simulink model "Load_Cell_Simulink"  (R2020a)
settings: Solver=VariableStepAuto  StartTime=0.0  StopTime=10  RelTol=1e-3
libraries: fl_lib x19, ee_lib x12, nesl_utility x7, simulink x1
settings Model: Creator=parsa  LastModifiedBy=parsa

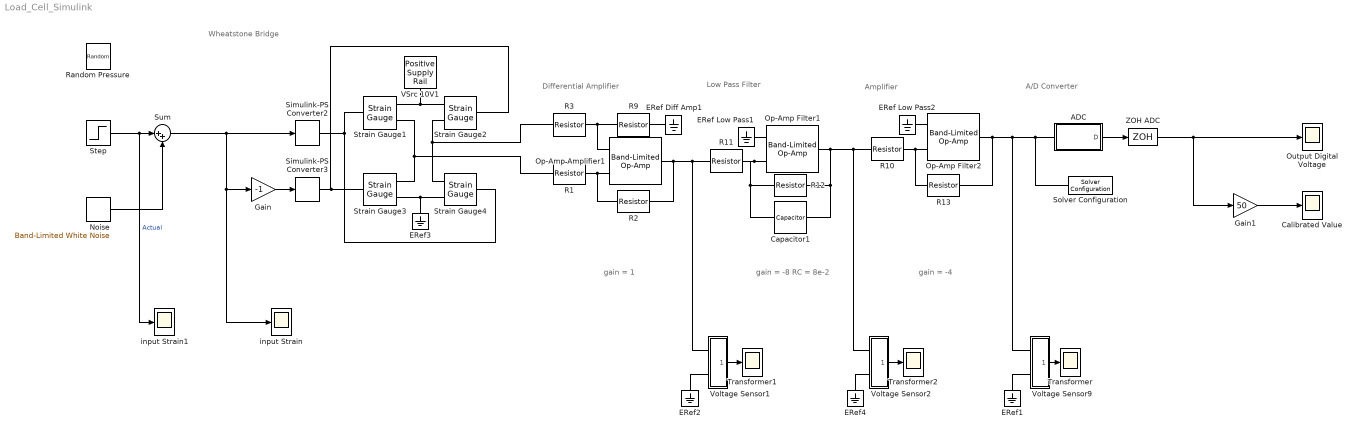
== system Load_Cell_Simulink ==
  note: A/D Converter
  note: Amplifier
  note: gain = -8
      | RC = 8e-2
  note: Low Pass Filter
  note: Wheatstone Bridge
  note: gain = 1
  note: Differential Amplifier
  note: gain = -4
  ADC : Subsystem  mask(ADC){N=24, vmax=9, ileak=1e-9, C=10e-12}
      mask prompts: N "Number of bits"; vmax "Input voltage for max output (V)"; ileak "Leakage current (A)"; C "Pin capacitance (F)"
      mask help: Simplified analog-to-digital converter
  Calibrated Value : Scope
  Capacitor1 : ee_lib/Passive/Capacitor  cap_option=0  c=10e-6 F  Cvec=[ 1e-5 1e-6 ] F  Vvec=[ 0 10 ] V  CV_table_symmetry=1  f_vec=[1, 10] kHz  DFext_vec=[.8, 1.2]  C_tol=5  enable_C_tol=0  tol_distribution=1  nSigma=4  r=1e-6 Ohm  g=0 1/Ohm  averaging_period=0 s  enable_operating_limits=0  operating_limit_action=2  max_working_voltage_range=[ -25 25 ] V  power_rating=1 W  enable_faults=0  fault_action=1  Cscale_faulted=100  R_faulted=0.001 Ohm  G_faulted=0 1/Ohm  tau_fault=0.001 s  enable_temporal_fault=0  t_fault=1 s  enable_behavioral_fault=0  max_permissible_voltage_range=[ -100 100 ] V  t_fail_on_voltage=1 s  i_specify=off  i_priority=None  i=0 A  i_nominal_specify=off  i_nominal_unit=A  i_nominal_value=1  v_specify=off  v_priority=None  v=0 V  v_nominal_specify=off  v_nominal_unit=V  v_nominal_value=1  vc_specify=on  vc_priority=High  vc=0 V  vc_nominal_specify=off  vc_nominal_unit=V  vc_nominal_value=1
  ERef Diff Amp1 : fl_lib/Electrical/Electrical Elements/Electrical Reference
      settings: SourceProductBaseCode=MT,SS
  ERef Low Pass1 : fl_lib/Electrical/Electrical Elements/Electrical Reference
      settings: SourceProductBaseCode=MT,SS
  ERef Low Pass2 : fl_lib/Electrical/Electrical Elements/Electrical Reference
      settings: SourceProductBaseCode=MT,SS
  ERef{1..4} (4 alike) : fl_lib/Electrical/Electrical Elements/Electrical Reference
  Gain : Gain  Gain=-1
  Gain1 : Gain  Gain=50
  Noise : simulink/Sources/Band-Limited White Noise  Cov=1e-10  Ts=0.001  seed=[23341]
  Op-Amp Amplifier1 : ee_lib/Integrated Circuits/Band-Limited Op-Amp  A=1000  Rin=1e+06 Ohm  Rout=100 Ohm  Vmin=-15 V  Vmax=15 V  Vdotmax=1000 V/s  f=1e5 Hz  V0=0 V
      settings: SourceProductBaseCode=PS
  Op-Amp Filter1 : ee_lib/Integrated Circuits/Band-Limited Op-Amp  A=1000  Rin=1e+06 Ohm  Rout=100 Ohm  Vmin=-15 V  Vmax=15 V  Vdotmax=1000 V/s  f=1e5 Hz  V0=0 V
      settings: SourceProductBaseCode=PS
  Op-Amp Filter2 : ee_lib/Integrated Circuits/Band-Limited Op-Amp  A=1000  Rin=1e+06 Ohm  Rout=100 Ohm  Vmin=-15 V  Vmax=15 V  Vdotmax=1000 V/s  f=1e5 Hz  V0=0 V
      settings: SourceProductBaseCode=PS
  Output Digital Voltage : Scope
  R{1..3,9} (4 alike) : fl_lib/Electrical/Electrical Elements/Resistor  R=10 kOhm  i_specify=off  i_priority=High  i=0 A  i_nominal_specify=off  i_nominal_unit=A  i_nominal_value=1  v_specify=off  v_priority=High  v=0 V  v_nominal_specify=off  v_nominal_unit=V  v_nominal_value=1
      settings: SourceProductBaseCode=MT,SS
  R10 : ee_lib/Passive/Resistor  R=1 kOhm  R_tol=5  enable_R_tol=0  tol_distribution=1  nSigma=4  enable_operating_limits=0  operating_limit_action=2  max_working_voltage=100 V  power_rating=1 W  enable_faults=0  fault_action=1  R_faulted=Inf Ohm  enable_temporal_fault=0  t_fault=1 s  enable_behavioral_fault=0  max_permissible_current=1 A  t_fail_on_current=1 s  noise_mode=0  sample_time=0.001 s  repeatability=1  auto_seed=2639802684  user_seed=0  Tdevice=25 degC  alpha=3.93e-3 1/K  Tmeas=25 degC  thermal_mass=100 J/K  power_derating_T1=70 degC  power_derating_T2=155 degC  operating_temperature_range_vec=[-50, 150] degC  temperature_specify=off  temperature_priority=High  temperature=298.15 K  temperature_nominal_specify=off  temperature_nominal_unit=K  temperature_nominal_value=1
  R11 : fl_lib/Electrical/Electrical Elements/Resistor  R=1 kOhm  i_specify=off  i_priority=High  i=0 A  i_nominal_specify=off  i_nominal_unit=A  i_nominal_value=1  v_specify=off  v_priority=High  v=0 V  v_nominal_specify=off  v_nominal_unit=V  v_nominal_value=1
      settings: SourceProductBaseCode=MT,SS
  R12 : ee_lib/Passive/Resistor  R=8 kOhm  R_tol=5  enable_R_tol=0  tol_distribution=1  nSigma=4  enable_operating_limits=0  operating_limit_action=2  max_working_voltage=100 V  power_rating=1 W  enable_faults=0  fault_action=1  R_faulted=Inf Ohm  enable_temporal_fault=0  t_fault=1 s  enable_behavioral_fault=0  max_permissible_current=1 A  t_fail_on_current=1 s  noise_mode=0  sample_time=0.001 s  repeatability=1  auto_seed=47154843  user_seed=0  Tdevice=25 degC  alpha=3.93e-3 1/K  Tmeas=25 degC  thermal_mass=100 J/K  power_derating_T1=70 degC  power_derating_T2=155 degC  operating_temperature_range_vec=[-50, 150] degC  temperature_specify=off  temperature_priority=High  temperature=298.15 K  temperature_nominal_specify=off  temperature_nominal_unit=K  temperature_nominal_value=1
  R13 : ee_lib/Passive/Resistor  R=4 kOhm  R_tol=5  enable_R_tol=0  tol_distribution=1  nSigma=4  enable_operating_limits=0  operating_limit_action=2  max_working_voltage=100 V  power_rating=1 W  enable_faults=0  fault_action=1  R_faulted=Inf Ohm  enable_temporal_fault=0  t_fault=1 s  enable_behavioral_fault=0  max_permissible_current=1 A  t_fail_on_current=1 s  noise_mode=0  sample_time=0.001 s  repeatability=1  auto_seed=2462134598  user_seed=0  Tdevice=25 degC  alpha=3.93e-3 1/K  Tmeas=25 degC  thermal_mass=100 J/K  power_derating_T1=70 degC  power_derating_T2=155 degC  operating_temperature_range_vec=[-50, 150] degC  temperature_specify=off  temperature_priority=High  temperature=298.15 K  temperature_nominal_specify=off  temperature_nominal_unit=K  temperature_nominal_value=1
  "Random Pressure " : UniformRandomNumber  Minimum=0  Maximum=1e-4  SampleTime=2
  Simulink-PS Converter2 : nesl_utility/Simulink-PS Converter  PhysicalDomain=network_engine_domain  SubClassName=ps_input  LeftPortType=input  RightPortType=output  PseudoPeriodic=off  Frequencies=[]  NoiseDistribution=none  NoiseParameters=[]  Unit=1  AffineConversion=off  FilteringAndDerivatives=zero  SimscapeFilterOrder=1  InputFilterTimeConstant=.001  UdotUserProvided=0
      settings: SourceProductBaseCode=MT,SS
  Simulink-PS Converter3 : nesl_utility/Simulink-PS Converter  PhysicalDomain=network_engine_domain  SubClassName=ps_input  LeftPortType=input  RightPortType=output  PseudoPeriodic=off  Frequencies=[]  NoiseDistribution=none  NoiseParameters=[]  Unit=1  AffineConversion=off  FilteringAndDerivatives=zero  SimscapeFilterOrder=1  InputFilterTimeConstant=.001  UdotUserProvided=0
      settings: SourceProductBaseCode=MT,SS
  Solver Configuration : nesl_utility/Solver Configuration  PhysicalDomain=network_engine_domain  SubClassName=solver  LeftPortType=input  RightPortType=generic  Tones=[]  Harmonics=[]  SimulateNoise=off  Profile=off  UseLocalSampling=off  EnableSwitchedLinearOptims=on  FrequencyDomain=off  UseCCode=off  RelTol=0.001  AbsTol=1e-06  MinStep=1e-09  ToWorkspace=off  RevertToSquareIcSolve=off  NumHomotopyIterations=100  PhasorMode=off  PhasorModeNumHarmonics=1  DoDC=off  ResidualTolerance=1e-09  UseLocalSolver=off  LocalSolverChoice=NE_BACKWARD_EULER_ADVANCER  LocalSolverSampleTime=0.001  DoFixedCost=off  MaxNonlinIter=3  MaxModeIter=2  LinearAlgebra=Sparse  EquationFormulation=NE_TIME_EF  DelaysMemoryBudget=1024  AutomaticFiltering=on  FilteringTimeConstant=0.001  PartitionStorageMethod=AS_NEEDED  PartitionMemoryBudget=1024  PartitionMethod=FAST
  Step : Step  After=1e-4  SampleTime=0
  Strain Gauge{1..4} (4 alike) : ee_lib/Sensors & Transducers/Strain Gauge  R=100 Ohm  K=2
      settings: SourceProductBaseCode=PS  InternalSimscapePortConfiguration="{\"Bottom\":[],\"Left\":[{\"id\":\"E\",\"label\":\"E\",\"type\":\"input\"}],\"Right\":[{\"id\":\"p\",\"label\":\"+\",\"type\":\"foundation.electrical.electrical\"},{\"id\":\"n\",\"label\":\"-\",\"type\":\"foundation.electrical.electrical\"}],\"Top\":[]}"
  Sum : Sum  Inputs=|++
  Transformer : Scope
  Transformer1 : Scope
  Transformer2 : Scope
  VSrc 10V1 : ee_lib/Sources/Positive Supply Rail  v0=9 V
      settings: SourceProductBaseCode=PS  InternalSimscapePortConfiguration="{\"Bottom\":[],\"Left\":[],\"Right\":[{\"id\":\"p\",\"label\":\"\",\"type\":\"foundation.electrical.electrical\"}],\"Top\":[]}"
  Voltage Sensor1 : Subsystem
  Voltage Sensor2 : Subsystem
  Voltage Sensor9 : Subsystem
  ZOH ADC : ZeroOrderHold  SampleTime=0.01
  input Strain : Scope
  input Strain1 : Scope
  wires:
  Gain/1 -> Simulink-PS Converter3/1
  ADC/1(D) -> ZOH ADC/1
  Voltage Sensor9/1(V) -> Transformer/1
  Voltage Sensor1/1(V) -> Transformer1/1
  Voltage Sensor2/1(V) -> Transformer2/1
  ZOH ADC/1 -> Gain1/1, Output Digital Voltage/1
  Gain1/1 -> Calibrated Value/1
  Noise/1 -> Sum/2
  Step/1 -> input Strain1/1, Sum/1  "Actual"
  Sum/1 -> input Strain/1, Gain/1, Simulink-PS Converter2/1
  connections:
  Op-Amp Filter2/LConn2 -- R10/RConn1 -- R13/LConn1
  Strain Gauge4/RConn2 -- Strain Gauge3/RConn2 -- ERef3/LConn1
  R3/LConn1 -- Strain Gauge4/RConn1 -- Strain Gauge2/RConn2
  Strain Gauge3/LConn1 -- Strain Gauge2/LConn1 -- Simulink-PS Converter3/RConn1
  R2/LConn1 -- Op-Amp Amplifier1/LConn2 -- R1/RConn1
  R1/LConn1 -- Strain Gauge1/RConn2 -- Strain Gauge3/RConn1
  Op-Amp Filter2/RConn1 -- R13/RConn1 -- Voltage Sensor9/LConn1 -- ADC/LConn1 -- Solver Configuration/RConn1
  Capacitor1/LConn1 -- R12/LConn1 -- R11/RConn1 -- Op-Amp Filter1/LConn2
  Capacitor1/RConn1 -- R12/RConn1 -- R10/LConn1 -- Voltage Sensor2/LConn1 -- Op-Amp Filter1/RConn1
  R2/RConn1 -- R11/LConn1 -- Voltage Sensor1/LConn1 -- Op-Amp Amplifier1/RConn1
  Strain Gauge1/RConn1 -- Strain Gauge2/RConn1 -- VSrc 10V1/RConn1
  Strain Gauge4/LConn1 -- Simulink-PS Converter2/RConn1 -- Strain Gauge1/LConn1
  R9/LConn1 -- R3/RConn1 -- Op-Amp Amplifier1/LConn1
  ERef Low Pass2/LConn1 -- Op-Amp Filter2/LConn1
  ERef Low Pass1/LConn1 -- Op-Amp Filter1/LConn1
  ERef Diff Amp1/LConn1 -- R9/RConn1
  ERef1/LConn1 -- Voltage Sensor9/LConn2
  ERef2/LConn1 -- Voltage Sensor1/LConn2
  ERef4/LConn1 -- Voltage Sensor2/LConn2

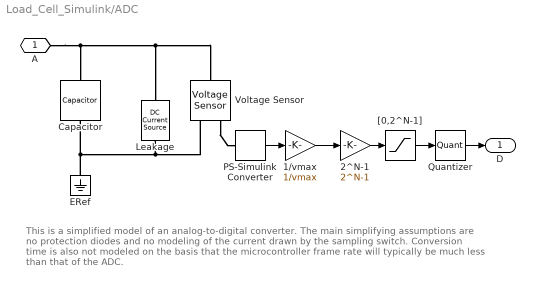
== system Load_Cell_Simulink/ADC ==
  note: This is a simplified model of an analog-to-digital converter. The main simplifying assumptions
      | are no protection diodes and no modeling of the current drawn by the sampling switch.
      | Conversion time is also not modeled on the basis that the microcontroller frame rate will
      | typically be much less than that of the ADC.
  1/vmax : Gain  Gain=1/vmax
  2^N-1 : Gain  Gain=2^N-1
  Capacitor : fl_lib/Electrical/Electrical Elements/Capacitor  c=1e-6 F  r=1e-6 Ohm  g=0 1/Ohm  i_specify=off  i_priority=High  i=0 A  i_nominal_specify=off  i_nominal_unit=A  i_nominal_value=1  v_specify=off  v_priority=High  v=0 V  v_nominal_specify=off  v_nominal_unit=V  v_nominal_value=1  vc_specify=on  vc_priority=High  vc=0 V  vc_nominal_specify=off  vc_nominal_unit=V  vc_nominal_value=1
      settings: SourceProductBaseCode=MT,SS
  ERef : fl_lib/Electrical/Electrical Elements/Electrical Reference
      settings: SourceProductBaseCode=MT,SS
  Leakage : fl_lib/Electrical/Electrical Sources/DC Current Source  i0=ileak A
      settings: SourceProductBaseCode=MT,SS  InternalSimscapePortConfiguration="{\"Bottom\":[],\"Left\":[{\"id\":\"p\",\"label\":\"\",\"type\":\"foundation.electrical.electrical\"}],\"Right\":[{\"id\":\"n\",\"label\":\"\",\"type\":\"foundation.electrical.electrical\"}],\"Top\":[]}"
  PS-Simulink Converter : nesl_utility/PS-Simulink Converter  PhysicalDomain=network_engine_domain  SubClassName=ps_output  LeftPortType=input  RightPortType=output  PseudoPeriodic=off  Frequencies=[]  Unit=V  AffineConversion=off
      settings: SourceProductBaseCode=MT,SS
  Quantizer : Quantizer
  Voltage Sensor : fl_lib/Electrical/Electrical Sensors/Voltage Sensor
      settings: SourceProductBaseCode=MT,SS
  "[0,2^N-1]" : Saturate  UpperLimit=2^N-1  LowerLimit=0
  A : PMIOPort  Side=Left
  D : Outport  VectorParamsAs1DForOutWhenUnconnected=off
  wires:
  1/vmax/1 -> 2^N-1/1
  2^N-1/1 -> "[0,2^N-1]"/1
  "[0,2^N-1]"/1 -> Quantizer/1
  Quantizer/1 -> D/1
  PS-Simulink Converter/1 -> 1/vmax/1
  connections:
  A/RConn1 -- Voltage Sensor/LConn1 -- Leakage/RConn1 -- Capacitor/LConn1
  ERef/LConn1 -- Voltage Sensor/RConn2 -- Leakage/LConn1 -- Capacitor/RConn1
  Voltage Sensor/RConn1 -- PS-Simulink Converter/LConn1

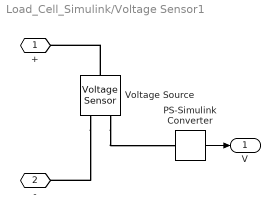
== system Load_Cell_Simulink/Voltage Sensor1 ==
  PS-Simulink Converter : nesl_utility/PS-Simulink Converter  PhysicalDomain=network_engine_domain  SubClassName=ps_output  LeftPortType=input  RightPortType=output  PseudoPeriodic=off  Frequencies=[]  Unit=1  AffineConversion=off
  Voltage Source : fl_lib/Electrical/Electrical Sensors/Voltage Sensor
  + : PMIOPort  Side=Left
  - : PMIOPort  Port=2  Side=Left
  V : Outport
  wires:
  PS-Simulink Converter/1 -> V/1
  connections:
  Voltage Source/RConn2 -- -/RConn1
  Voltage Source/LConn1 -- +/RConn1
  Voltage Source/RConn1 -- PS-Simulink Converter/LConn1

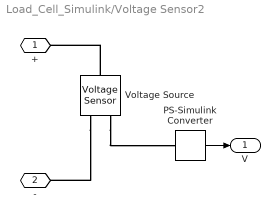
== system Load_Cell_Simulink/Voltage Sensor2 ==
  PS-Simulink Converter : nesl_utility/PS-Simulink Converter  PhysicalDomain=network_engine_domain  SubClassName=ps_output  LeftPortType=input  RightPortType=output  PseudoPeriodic=off  Frequencies=[]  Unit=1  AffineConversion=off
  Voltage Source : fl_lib/Electrical/Electrical Sensors/Voltage Sensor
  + : PMIOPort  Side=Left
  - : PMIOPort  Port=2  Side=Left
  V : Outport
  wires:
  PS-Simulink Converter/1 -> V/1
  connections:
  Voltage Source/RConn2 -- -/RConn1
  Voltage Source/LConn1 -- +/RConn1
  Voltage Source/RConn1 -- PS-Simulink Converter/LConn1

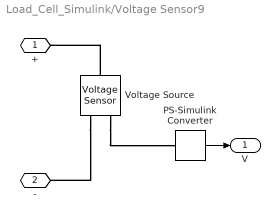
== system Load_Cell_Simulink/Voltage Sensor9 ==
  PS-Simulink Converter : nesl_utility/PS-Simulink Converter  PhysicalDomain=network_engine_domain  SubClassName=ps_output  LeftPortType=input  RightPortType=output  PseudoPeriodic=off  Frequencies=[]  Unit=1  AffineConversion=off
  Voltage Source : fl_lib/Electrical/Electrical Sensors/Voltage Sensor
  + : PMIOPort  Side=Left
  - : PMIOPort  Port=2  Side=Left
  V : Outport
  wires:
  PS-Simulink Converter/1 -> V/1
  connections:
  Voltage Source/RConn2 -- -/RConn1
  Voltage Source/LConn1 -- +/RConn1
  Voltage Source/RConn1 -- PS-Simulink Converter/LConn1
